simulink model "currentloop_pi_test"  (R2023b)
settings: Solver=FixedStepAuto  StartTime=0.0  StopTime=simcfg.stop_time  FixedStep=simcfg.Ts_plant  RelTol=1e-3
InitFcn:
  | motor_control_params
undefined symbols (not defined in the file or in its folder): control, inverter, motor, simcfg
libraries: mcbplantlib x1, autolibpmsmexterior x1
settings Model: Creator=user  LastModifiedBy=user

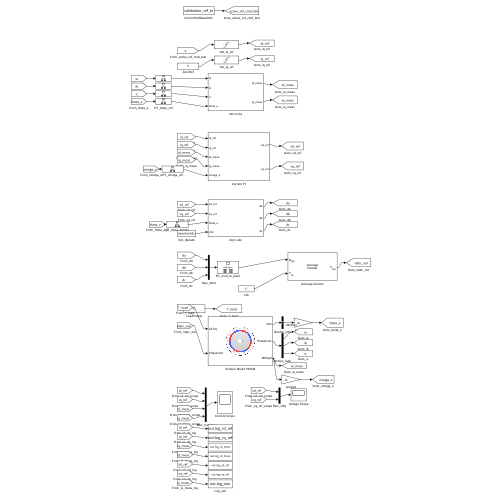
[thumbnail: Simulink's stored preview of the top-level diagram]
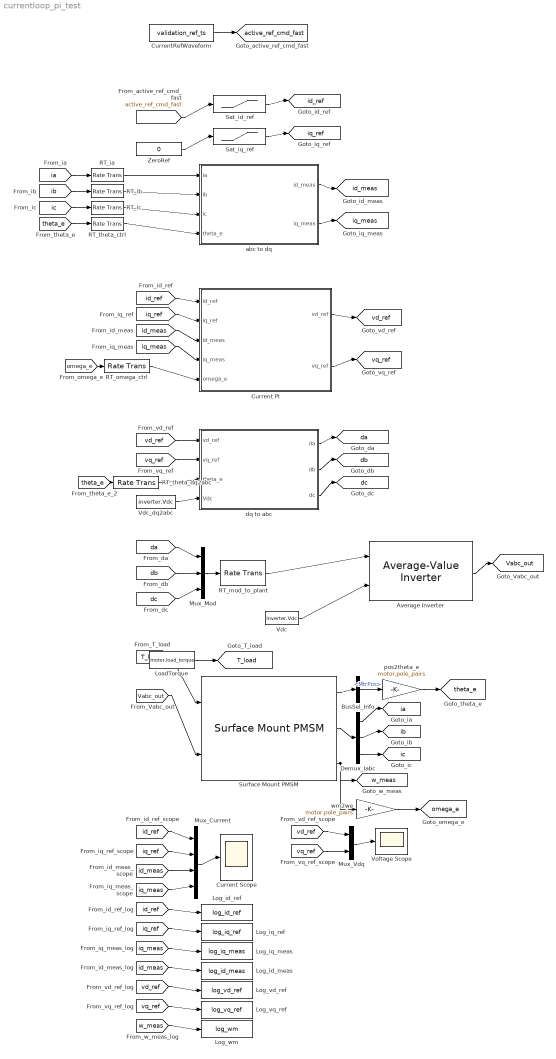
== system currentloop_pi_test ==
  Average Inverter : mcbplantlib/Average-Value Inverter
  BusSel_Info : BusSelector  OutputSignals=MtrPos
  Current PI : Subsystem
  Current Scope : Scope
  CurrentRefWaveform : FromWorkspace  VariableName=validation_ref_ts
  Demux_Iabc : Demux  Outputs=3
  LoadTorque : Constant  Value=motor.load_torque
  Log_id_meas : ToWorkspace  VariableName=log_id_meas  SaveFormat=Timeseries  SampleTime=-1
  Log_id_ref : ToWorkspace  VariableName=log_id_ref  SaveFormat=Timeseries  SampleTime=-1
  Log_iq_meas : ToWorkspace  VariableName=log_iq_meas  SaveFormat=Timeseries  SampleTime=-1
  Log_iq_ref : ToWorkspace  VariableName=log_iq_ref  SaveFormat=Timeseries  SampleTime=-1
  Log_vd_ref : ToWorkspace  VariableName=log_vd_ref  SaveFormat=Timeseries  SampleTime=-1
  Log_vq_ref : ToWorkspace  VariableName=log_vq_ref  SaveFormat=Timeseries  SampleTime=-1
  Log_wm : ToWorkspace  VariableName=log_wm  SaveFormat=Timeseries  SampleTime=-1
  Mux_Current : Mux
  Mux_Mod : Mux  Inputs=3
  Mux_Vdq : Mux  Inputs=2
  RT_ia : RateTransition  OutPortSampleTime=simcfg.Ts_ctrl
  RT_ib : RateTransition  OutPortSampleTime=simcfg.Ts_ctrl
  RT_ic : RateTransition  OutPortSampleTime=simcfg.Ts_ctrl
  RT_mod_to_plant : RateTransition  OutPortSampleTime=simcfg.Ts_plant
  RT_omega_ctrl : RateTransition  OutPortSampleTime=simcfg.Ts_ctrl
  RT_theta_ctrl : RateTransition  OutPortSampleTime=simcfg.Ts_ctrl
  RT_theta_dq2abc : RateTransition  OutPortSampleTime=simcfg.Ts_ctrl
  Sat_id_ref : Saturate  UpperLimit=control.iq_ref_limit  LowerLimit=-control.iq_ref_limit
  Sat_iq_ref : Saturate  UpperLimit=control.iq_ref_limit  LowerLimit=-control.iq_ref_limit
  Surface Mount PMSM : autolibpmsmexterior/Surface Mount PMSM  port_config=Torque  sim_type=Discrete  Ts=simcfg.Ts_plant  P=motor.pole_pairs  Rs=motor.Rs  Ldq_=motor.Ld  KConstText=Permanent flux linkage constant (lambda_pm):  lambda_pm=motor.psi_f  Ke=159.9771  Kt=1.323  mechanical=[motor.J, motor.B, 0]  idq0=[0 0]  theta_init=0  omega_init=0  KConst=motor.psi_f  lambda_pm_calc=motor.psi_f  RefBlkName='autolibpmsmexterior/Surface Mount PMSM'  aMode=5  Ldq="[0.0017      0.0017]"
  Vdc : Constant  Value=inverter.Vdc
  Vdc_dq2abc : Constant  Value=inverter.Vdc
  Voltage Scope : Scope
  ZeroRef : Constant  Value=0
  abc to dq : Subsystem
  dq to abc : Subsystem
  pos2theta_e : Gain  Gain=motor.pole_pairs
  wm2we : Gain  Gain=motor.pole_pairs
  tag scope: T_load=global, Vabc_out=global, active_ref_cmd_fast=global, da=global, db=global, dc=global, ia=global, ib=global, ic=global, id_meas=global, id_ref=global, iq_meas=global, iq_ref=global, omega_e=global, theta_e=global, vd_ref=global, vq_ref=global, w_meas=global
  wires:
  CurrentRefWaveform/1 -> [active_ref_cmd_fast]
  [active_ref_cmd_fast] -> Sat_id_ref/1
  ZeroRef/1 -> Sat_iq_ref/1
  Sat_id_ref/1 -> [id_ref]
  Sat_iq_ref/1 -> [iq_ref]
  [ia] -> RT_ia/1
  [ib] -> RT_ib/1
  [ic] -> RT_ic/1
  [theta_e] -> RT_theta_ctrl/1
  RT_ia/1 -> abc to dq/1(ia)
  RT_ib/1 -> abc to dq/2(ib)
  RT_ic/1 -> abc to dq/3(ic)
  RT_theta_ctrl/1 -> abc to dq/4(theta_e)
  abc to dq/1(id_meas) -> [id_meas]
  abc to dq/2(iq_meas) -> [iq_meas]
  [omega_e] -> RT_omega_ctrl/1
  [id_ref] -> Current PI/1(id_ref)
  [iq_ref] -> Current PI/2(iq_ref)
  [id_meas] -> Current PI/3(id_meas)
  [iq_meas] -> Current PI/4(iq_meas)
  RT_omega_ctrl/1 -> Current PI/5(omega_e)
  Current PI/1(vd_ref) -> [vd_ref]
  Current PI/2(vq_ref) -> [vq_ref]
  [theta_e] -> RT_theta_dq2abc/1
  [vd_ref] -> dq to abc/1(vd_ref)
  [vq_ref] -> dq to abc/2(vq_ref)
  RT_theta_dq2abc/1 -> dq to abc/3(theta_e)
  Vdc_dq2abc/1 -> dq to abc/4(Vdc)
  dq to abc/1(da) -> [da]
  dq to abc/2(db) -> [db]
  dq to abc/3(dc) -> [dc]
  [da] -> Mux_Mod/1
  [db] -> Mux_Mod/2
  [dc] -> Mux_Mod/3
  Mux_Mod/1 -> RT_mod_to_plant/1
  RT_mod_to_plant/1 -> Average Inverter/1
  Vdc/1 -> Average Inverter/2
  Average Inverter/1 -> [Vabc_out]
  LoadTorque/1 -> [T_load]
  [T_load] -> Surface Mount PMSM/1
  [Vabc_out] -> Surface Mount PMSM/2
  Surface Mount PMSM/1 -> BusSel_Info/1
  BusSel_Info/1 -> pos2theta_e/1  "<MtrPos>"
  pos2theta_e/1 -> [theta_e]
  Surface Mount PMSM/2 -> Demux_Iabc/1
  Demux_Iabc/1 -> [ia]
  Demux_Iabc/2 -> [ib]
  Demux_Iabc/3 -> [ic]
  Surface Mount PMSM/3 -> [w_meas], wm2we/1
  wm2we/1 -> [omega_e]
  [id_ref] -> Mux_Current/1
  [iq_ref] -> Mux_Current/2
  [id_meas] -> Mux_Current/3
  [iq_meas] -> Mux_Current/4
  Mux_Current/1 -> Current Scope/1
  [vd_ref] -> Mux_Vdq/1
  [vq_ref] -> Mux_Vdq/2
  Mux_Vdq/1 -> Voltage Scope/1
  [id_ref] -> Log_id_ref/1
  [iq_ref] -> Log_iq_ref/1
  [iq_meas] -> Log_iq_meas/1
  [id_meas] -> Log_id_meas/1
  [vd_ref] -> Log_vd_ref/1
  [vq_ref] -> Log_vq_ref/1
  [w_meas] -> Log_wm/1

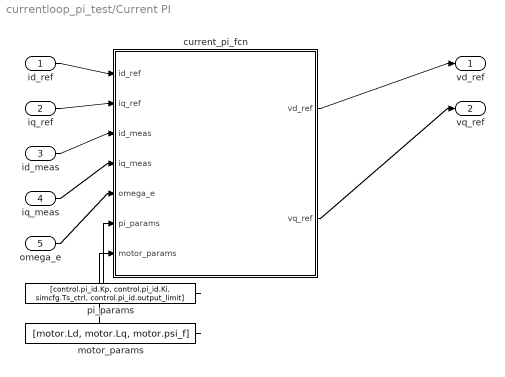
== system currentloop_pi_test/Current PI ==
  id_ref : Inport
  iq_ref : Inport  Port=2
  id_meas : Inport  Port=3
  iq_meas : Inport  Port=4
  omega_e : Inport  Port=5
  current_pi_fcn : MATLAB Function  TreatAsAtomicUnit=on
  motor_params : Constant  Value=[motor.Ld, motor.Lq, motor.psi_f]
  pi_params : Constant  Value=[control.pi_id.Kp, control.pi_id.Ki, simcfg.Ts_ctrl, control.pi_id.output_limit]
  vd_ref : Outport
  vq_ref : Outport  Port=2
  wires:
  id_ref/1 -> current_pi_fcn/1(id_ref)
  iq_ref/1 -> current_pi_fcn/2(iq_ref)
  id_meas/1 -> current_pi_fcn/3(id_meas)
  iq_meas/1 -> current_pi_fcn/4(iq_meas)
  omega_e/1 -> current_pi_fcn/5(omega_e)
  pi_params/1 -> current_pi_fcn/6(pi_params)
  motor_params/1 -> current_pi_fcn/7(motor_params)
  current_pi_fcn/1(vd_ref) -> vd_ref/1
  current_pi_fcn/2(vq_ref) -> vq_ref/1

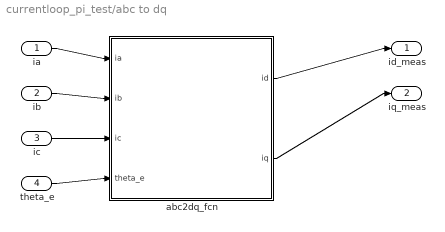
== system currentloop_pi_test/abc to dq ==
  ia : Inport
  ib : Inport  Port=2
  ic : Inport  Port=3
  theta_e : Inport  Port=4
  abc2dq_fcn : MATLAB Function  TreatAsAtomicUnit=on
  id_meas : Outport
  iq_meas : Outport  Port=2
  wires:
  ia/1 -> abc2dq_fcn/1(ia)
  ib/1 -> abc2dq_fcn/2(ib)
  ic/1 -> abc2dq_fcn/3(ic)
  theta_e/1 -> abc2dq_fcn/4(theta_e)
  abc2dq_fcn/1(id) -> id_meas/1
  abc2dq_fcn/2(iq) -> iq_meas/1

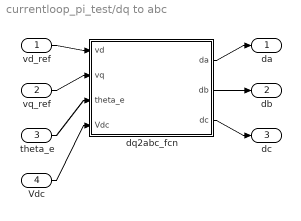
== system currentloop_pi_test/dq to abc ==
  vd_ref : Inport
  vq_ref : Inport  Port=2
  theta_e : Inport  Port=3
  Vdc : Inport  Port=4
  dq2abc_fcn : MATLAB Function  TreatAsAtomicUnit=on
  da : Outport
  db : Outport  Port=2
  dc : Outport  Port=3
  wires:
  vd_ref/1 -> dq2abc_fcn/1(vd)
  vq_ref/1 -> dq2abc_fcn/2(vq)
  theta_e/1 -> dq2abc_fcn/3(theta_e)
  Vdc/1 -> dq2abc_fcn/4(Vdc)
  dq2abc_fcn/1(da) -> da/1
  dq2abc_fcn/2(db) -> db/1
  dq2abc_fcn/3(dc) -> dc/1

== matlab function currentloop_pi_test/Current PI/current_pi_fcn ==
  data: id_ref input; vd_ref output; iq_ref input; id_meas input; iq_meas input; omega_e input; pi_params input; motor_params input; vq_ref output
function [vd_ref, vq_ref] = current_pi_fcn(id_ref, iq_ref, id_meas, iq_meas, omega_e, pi_params, motor_params)
% Discrete PI current controller with cross-coupling decoupling
% pi_params    = [Kp, Ki, Ts, output_limit]
% motor_params = [Ld, Lq, psi_f]
persistent int_d int_q
if isempty(int_d)
    int_d = 0;
    int_q = 0;
end
Kp = pi_params(1); Ki = pi_params(2); Ts = pi_params(3); lim = pi_params(4);
Ld = motor_params(1); Lq = motor_params(2); psi_f = motor_params(3);

% d-axis PI
err_d = id_ref - id_meas;
int_d = int_d + Ki * Ts * err_d;
int_d = max(-lim, min(lim, int_d));
vd_pi = Kp * err_d + int_d;

% q-axis PI
err_q = iq_ref - iq_meas;
int_q = int_q + Ki * Ts * err_q;
int_q = max(-lim, min(lim, int_q));
vq_pi = Kp * err_q + int_q;

% Cross-coupling decoupling
vd_dec = -omega_e * Lq * iq_meas;
vq_dec = omega_e * (Ld * id_meas + psi_f);

% Output
vd_ref = vd_pi + vd_dec;
vq_ref = vq_pi + vq_dec;

== matlab function currentloop_pi_test/abc to dq/abc2dq_fcn ==
  data: ia input; id output; ib input; ic input; theta_e input; iq output
function [id, iq] = abc2dq_fcn(ia, ib, ic, theta_e)
% abc to dq: Clarke + Park transform

% 1. Clarke: abc -> alpha-beta (equal-amplitude)
i_alpha = (2/3) * (ia - 0.5*ib - 0.5*ic);
i_beta  = (2/3) * (sqrt(3)/2*ib - sqrt(3)/2*ic);

% 2. Park: alpha-beta -> dq
id = i_alpha * cos(theta_e) + i_beta * sin(theta_e);
iq = -i_alpha * sin(theta_e) + i_beta * cos(theta_e);

== matlab function currentloop_pi_test/dq to abc/dq2abc_fcn ==
  data: vd input; da output; vq input; theta_e input; Vdc input; db output; dc output
function [da, db, dc] = dq2abc_fcn(vd, vq, theta_e, Vdc)
% dq -> 占空比: 逆Park + 逆Clarke + SVPWM + 归一化

% 1. 逆Park: dq -> alpha-beta
v_alpha = vd * cos(theta_e) - vq * sin(theta_e);
v_beta  = vd * sin(theta_e) + vq * cos(theta_e);

% 2. 逆Clarke: alpha-beta -> abc
va = v_alpha;
vb = -0.5 * v_alpha + sqrt(3)/2 * v_beta;
vc = -0.5 * v_alpha - sqrt(3)/2 * v_beta;

% 3. SVPWM零序注入
v_max = max(max(va, vb), vc);
v_min = min(min(va, vb), vc);
v_n0  = -0.5 * (v_max + v_min);
va = va + v_n0;
vb = vb + v_n0;
vc = vc + v_n0;

%% 4. 占空比 [0,1]
da = va / Vdc + 0.5;
db = vb / Vdc + 0.5;
dc = vc / Vdc + 0.5;
